simulink model "testbed_overall"  (R2022a)
settings: Solver=ode3  StartTime=0.0  StopTime=8  FixedStep=Ts  RelTol=1e-3
InitFcn:
  | f = 60;
  | Sb = 1e6; % base power
  | Vb_S = 13.2e3*sqrt(2)/sqrt(3);% secondary side base voltage phase to ground
  | Ib_S =Sb/Vb_S; % secondary side base current
  | Vb_P = 400*sqrt(2)/sqrt(3); % primary side base V
  | Ib_P = Sb/Vb_P; % primary side base I
  | Zb = ((400)^2)/Sb; % primary side base impedance
  | Zs = ((13.2e3)^2)/Sb; % secondary side base impedance
  | Zt = 0.02+1i*0.0721; % transformer impedance
  | Vg = 1;
  | P = 0.5;
  | Q = 0.5;
  | S = P+1i*Q;
  | I3 = conj(S/Vg);
  | V3 = Vg+I3*Zt; % pcc voltage in S side
  | % Vpcc = V3*Vb_S/Vb_P; % P side
  | Vpcc = V3;
  | R1 = 0.001/Zb;
  | L1 = (1i*120*pi*46e-6)/Zb; % impedacne ZL1
  | C1 = -(1i/(120*pi*3*444e-6))/Zb; %impedance ZC1
  | I2 = Vpcc/C1; % curreent going through the Capcitor
  | I1 = I2+I3;
  | V1 = Vpcc+I1*(R1+L1);
  | V = V1*Vb_P;
values from neighbouring files (symbols this model uses):
  ang_0 = 22*pi/180    (= 0.383972435439)    [GFM_initial.m]
  bc = w0*cf*zb1    (= 0.08034434716)    [GFM_initial.m]
  K1 = 1/0.05    (= 20)    [GFM_initial.m]
  K2 = 0.3    [GFM_initial.m]
  Ki_P = 25    [GFM_initial.m]
  ki_PLL = 1400    [GFM_initial.m]
  Ki_v = 40    [GFM_initial.m]
  Ki_vq = 10    [GFM_initial.m]
  kii = 3.2655    [GFM_initial.m]
  kiv = 40    [GFM_initial.m]
  Kp_P = 0.25    [GFM_initial.m]
  kp_PLL = 60    [GFM_initial.m]
  Kp_v = 0.4    [GFM_initial.m]
  Kp_vq = 1    [GFM_initial.m]
  kpi = 0.4758    [GFM_initial.m]
  kpv = 0.4    [GFM_initial.m]
  lg_real = xgrid_pu*zb2/w0    (= 0.369748763791)    [GFM_initial.m]
  rg_real = rgrid_pu*zb2    (= 13.9392)    [GFM_initial.m]
  Ts = 50e-6    (= 5e-05)    [GFM_initial.m]
  vb1 = vn1*sqrt(2/3)    [GFM_initial.m]
  w0 = 2*pi*f    (= 376.991118431)    [GFM_initial.m]
  xfpu = 2*pi*60*(46e-6)/0.16    (= 0.108384946549)    [GFM_initial.m]
undefined symbols (not defined in the file or in its folder): DiscIntNeverNeededParam
libraries: spsFirstOrderFilterLib x25, spsabctodq0Lib x13, spsPower3phInstantaneousLib x4, spsdq0toabcLib x4, spsThreePhaseVIMeasurementLib x4, spsThreePhaseSeriesRLCBranchLib x3, spsGroundLib x2, spsThreePhaseBreakerLib x2, spsSeriesRLCBranchLib x2, spsThreePhaseTransformerTwoWindingsLib x1, spsThreePhaseSeriesRLCLoadLib x1, spsThreePhaseParallelRLCBranchLib x1
settings Model: Creator=joshua  LastModifiedBy=PSCAD_FAN
settings SolverCC: AlgebraicLoopSolver=TrustRegion
settings DebuggingCC: UnconnectedInputMsg=warning  UnconnectedOutputMsg=warning  UnconnectedLineMsg=warning  SFMachineParentedDataDiag=warning  ArithmeticOperatorsInVariantConditions=warning
settings SFSimCC: CustomCodeUndefinedFunction=UseInterfaceOnly
settings RTWCC: DLArmComputeVersion=19.05
settings CodeAppCC: StateflowObjectComments=on
settings SimscapeCC: SimscapeNormalizeSystem=off

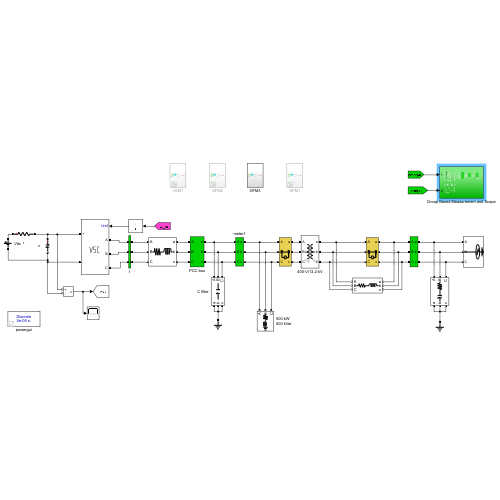
[thumbnail: Simulink's stored preview of the top-level diagram]
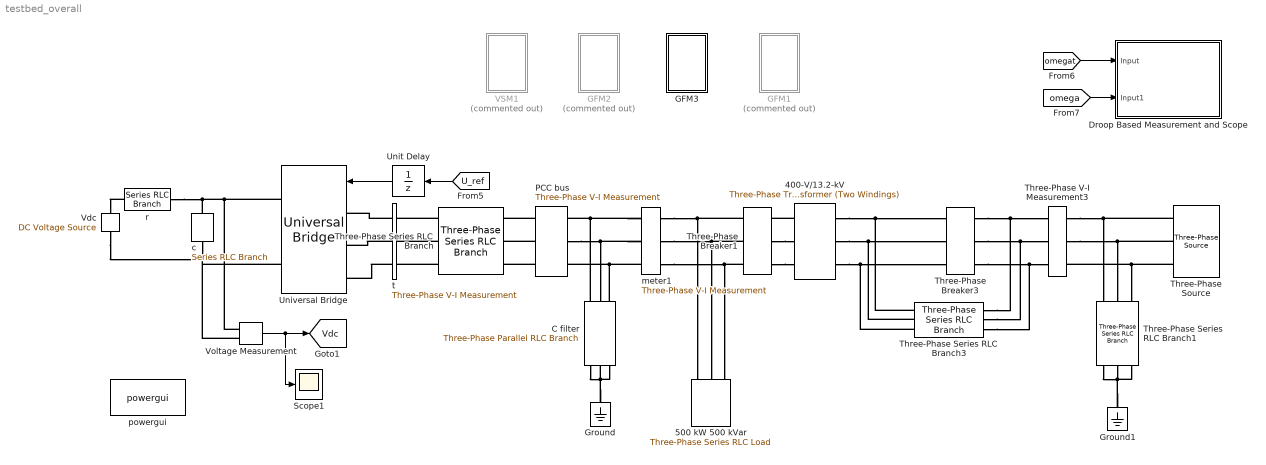
== system testbed_overall ==
  400-V/13.2-kV : spsThreePhaseTransformerTwoWindingsLib/Three-Phase Transformer (Two Windings)  Winding1Connection=Yg  Winding2Connection=Yg  CoreType=Three single-phase transformers  SetSaturation=off  Hysteresis=off  DataFile='hysteresis'  SetInitialFlux=off  Measurements=Winding voltages  UNITS=pu  NominalPower=[1e6 , 60 ]  Winding1=[400 0.01 0.0721/2]  Winding2=[13200 0.01 0.0721/2]  Rm=500  Lm=500  L0=0.50001  Saturation=[0 0;4.8989 1.0396;2041.2 1.3168]  InitialFluxes=[0.69306 -0.69306 0.60643]  BreakLoop=off  DiscreteSolver=Trapezoidal iterative  DataType=off  TransfoNumber=1
  500 kW 500 kVar : spsThreePhaseSeriesRLCLoadLib/Three-Phase Series RLC Load  LConnTagsString=A|B|C  Configuration=Y (grounded)  NominalVoltage=400  Vabc=[1e3 1e3 1e3]  Vabcp=[1e3 1e3 1e3]  NominalFrequency=f  UnbalancedPower=off  ActivePower=0.5*Sb  InductivePower=0.5*Sb  CapacitivePower=0  Pabc=[10e3 9e3 11e3]  QLabc=[100 90 110]  QCabc=[100 90 110]  Pabcp=[10e3 9e3 11e3]  QLabcp=[100 90 110]  QCabcp=[100 90 110]  Measurements=None  LoadType=constant Z
  C filter : spsThreePhaseParallelRLCBranchLib/Three-Phase Parallel RLC Branch  LConnTagsString=A|B|C  RConnTagsString=A|B|C  BranchType=C  Resistance=1  Inductance=1e-3  Capacitance=444e-6  Measurements=None
      settings: SourceProductBaseCode=PS
  Droop Based Measurement and Scope : Subsystem
  GFM1 : Subsystem  Commented=on
  GFM2 : Subsystem  Commented=on
  GFM3 : Subsystem
  Ground : spsGroundLib/Ground  LConnTagsString=a
  Ground1 : spsGroundLib/Ground  LConnTagsString=a
  PCC bus : spsThreePhaseVIMeasurementLib/Three-Phase V-I Measurement  VoltageMeasurement=phase-to-ground  SetLabelV=on  LabelV=Vpcc  Vpu=on  VpuLL=off  CurrentMeasurement=yes  SetLabelI=on  LabelI=Iconv  Ipu=on  Pbase=1e6  Vbase=400  OutputType=Complex  PhasorSimulation=off  PSBequivalent=0
  Scope1 : Scope
  Three-Phase Series RLC Branch : spsThreePhaseSeriesRLCBranchLib/Three-Phase Series RLC Branch  LConnTagsString=A|B|C  RConnTagsString=A|B|C  BranchType=RL  Resistance=0.001  Inductance=46e-6  Capacitance=1e-6  Measurements=None
  Three-Phase Series RLC Branch1 : spsThreePhaseSeriesRLCBranchLib/Three-Phase Series RLC Branch  LConnTagsString=A|B|C  RConnTagsString=A|B|C  BranchType=RC  Resistance=15  Inductance=1e-3  Capacitance=6.39e-6  Measurements=None
  Three-Phase Series RLC Branch3 : spsThreePhaseSeriesRLCBranchLib/Three-Phase Series RLC Branch  LConnTagsString=A|B|C  RConnTagsString=A|B|C  BranchType=RL  Resistance=rg_real  Inductance=lg_real  Capacitance=1e-6  Measurements=None
  Three-Phase V-I Measurement3 : spsThreePhaseVIMeasurementLib/Three-Phase V-I Measurement  VoltageMeasurement=phase-to-ground  SetLabelV=on  LabelV=Vabc  Vpu=on  VpuLL=off  CurrentMeasurement=yes  SetLabelI=on  LabelI=Ig  Ipu=on  Pbase=1e6  Vbase=13.2e3  OutputType=Complex  PhasorSimulation=off  PSBequivalent=0
  Three-Phase Breaker1 : spsThreePhaseBreakerLib/Three-Phase Breaker  InitialState=closed  SwitchA=on  SwitchB=on  SwitchC=on  SwitchTimes=[4,6]  External=off  BreakerResistance=0.0001  SnubberResistance=1e7  SnubberCapacitance=inf  Measurements=None
  Three-Phase Breaker3 : spsThreePhaseBreakerLib/Three-Phase Breaker  InitialState=closed  SwitchA=on  SwitchB=on  SwitchC=on  SwitchTimes=[2]  External=off  BreakerResistance=0.0001  SnubberResistance=1e7  SnubberCapacitance=inf  Measurements=None
  Three-Phase Source : spsThreePhaseSourceLib/Three-Phase Source  InternalConnection=Yg  VoltagePhases=off  Voltage=13.2e3  PhaseAngle=0  Voltage_phases=[25e3*0.5 25e3 25e3]/sqrt(3)  PhaseAngles_phases=[0 -120 +120]  Frequency=60  NonIdealSource=off  SpecifyImpedance=off  Resistance=0.8929  Inductance=16.58e-3  ShortCircuitLevel=100e6  BaseVoltage=25e3  XRratio=7  BusType=swing  Pref=10e3  Qref=0  Prefabc=[10e3, 10e3, 10e3]  Qrefabc=[0, 0, 0]  Qmin=-inf  Qmax=inf
  Unit Delay : UnitDelay  SampleTime=-1  HasFrameUpgradeWarning=on
  Universal Bridge : spsUniversalBridgeLib/Universal Bridge  Arms=3  SnubberResistance=1e5  SnubberCapacitance=inf  Device=Average-model based VSC  Ron=1e-3  Lon=0  ForwardVoltages="[  0  0  ]"  ForwardVoltage=0  GTOparameters=[ 10e-6 , 20e-6 ]  IGBTparameters=[ 1e-6 , 2e-6 ]  Measurements=None  Measurements_2=None  converterType=Rectifier
  VSM1 : Subsystem  Commented=on
  Vdc : spsDCVoltageSourceLib/DC Voltage Source  Amplitude=1025.6315  Measurements=None
  Voltage Measurement : spsVoltageMeasurementLib/Voltage Measurement  PhasorSimulation=off  OutputType=Complex  PSBequivalent=0
  c : spsSeriesRLCBranchLib/Series RLC Branch  LConnTagsString=__new0  RConnTagsString=__new0  BranchType=C  Resistance=0.05  Inductance=1e-3  SetiL0=off  InitialCurrent=0  Capacitance=0.04  Setx0=off  InitialVoltage=0  Measurements=Branch voltage
  meter1 : spsThreePhaseVIMeasurementLib/Three-Phase V-I Measurement  VoltageMeasurement=phase-to-ground  SetLabelV=on  LabelV=Vload  Vpu=on  VpuLL=off  CurrentMeasurement=yes  SetLabelI=on  LabelI=Iload  Ipu=on  Pbase=1e6  Vbase=400  OutputType=Complex  PhasorSimulation=off  PSBequivalent=0
  powergui : spspowerguiLib/powergui  Priority=1  SimulationMode=Discrete  SampleTime=50e-6  frequency=60  Iterations=50  frequencyindice=0  Pbase=100e6  ErrMax=1e-4  UnitsV=kV  UnitsW=MW  buscounter=0  FunctionMessages=off  echomessages=off  EnableUseOfTLC=off  CurrentSourceSwitches=off  DisableSnubberDevices=off  DisableRonSwitches=off  DisableVfSwitches=off  DisplayEquations=off  AutomaticDiscreteSolvers=off  SolverType=Tustin/Backward Euler (TBE)  Interpol=off  ExternalGateDelay=off  methode=off  Ts=100  x0status=blocks  SPID=on  SwTol=0  HookPort=off  NonlinearTolerance=1e-4  nMaxIteration=100  ContinueOnMaxIteration=off  RestoreLinks=warning  ResistiveCurrentMeasurement=off  Frange=[0:2:500]  Ylog=off  Xlog=on  ShowGrid=off  save=off  variable=ZData  structure=0  ZoomFFT=off  StartTime=0.0  cycles=1  DisplayStyle=1  fundamental=60  FreqAxis=off  MaxFrequency=1000  frequencyindicesteady=1  RmsSteady=1  display=off
  r : spsSeriesRLCBranchLib/Series RLC Branch  LConnTagsString=__new0  RConnTagsString=__new0  BranchType=R  Resistance=0.05  Inductance=1e-3  SetiL0=off  InitialCurrent=0  Capacitance=1e-6  Setx0=off  InitialVoltage=0  Measurements=None
  t : spsThreePhaseVIMeasurementLib/Three-Phase V-I Measurement  VoltageMeasurement=phase-to-ground  SetLabelV=on  LabelV=Vabc_o  Vpu=on  VpuLL=off  CurrentMeasurement=yes  SetLabelI=on  LabelI=Io  Ipu=on  Pbase=1e6  Vbase=400  OutputType=Complex  PhasorSimulation=off  PSBequivalent=0
  tag scope: Vdc=global
  wires:
  Voltage Measurement/1 -> Scope1/1, [Vdc]
  [U_ref] -> Unit Delay/1
  Unit Delay/1 -> Universal Bridge/1
  [omegat] -> Droop Based Measurement and Scope/1(Input)
  [omega] -> Droop Based Measurement and Scope/2(Input1)
  connections:
  Three-Phase Series RLC Branch1/RConn1 -- Three-Phase Series RLC Branch1/RConn3 -- Ground1/LConn1 -- Three-Phase Series RLC Branch1/RConn2
  PCC bus/RConn2 -- meter1/LConn2 -- C filter/LConn2
  Three-Phase V-I Measurement3/RConn2 -- Three-Phase Source/RConn2 -- Three-Phase Series RLC Branch1/LConn2
  Three-Phase Breaker1/LConn3 -- meter1/RConn3 -- 500 kW 500 kVar/LConn3
  Voltage Measurement/LConn1 -- Universal Bridge/RConn1 -- r/RConn1 -- c/LConn1
  c/RConn1 -- Universal Bridge/RConn2 -- Voltage Measurement/LConn2 -- Vdc/LConn1
  C filter/RConn2 -- C filter/RConn3 -- Ground/LConn1 -- C filter/RConn1
  C filter/LConn1 -- PCC bus/RConn1 -- meter1/LConn1
  Three-Phase V-I Measurement3/RConn1 -- Three-Phase Source/RConn1 -- Three-Phase Series RLC Branch1/LConn1
  Three-Phase Source/RConn3 -- Three-Phase V-I Measurement3/RConn3 -- Three-Phase Series RLC Branch1/LConn3
  400-V/13.2-kV/LConn1 -- Three-Phase Breaker1/RConn1
  r/LConn1 -- Vdc/RConn1
  Three-Phase Breaker1/RConn2 -- 400-V/13.2-kV/LConn2
  PCC bus/LConn3 -- Three-Phase Series RLC Branch/RConn3
  PCC bus/LConn1 -- Three-Phase Series RLC Branch/RConn1
  Three-Phase Series RLC Branch/LConn1 -- t/RConn1
  Three-Phase Breaker1/RConn3 -- 400-V/13.2-kV/LConn3
  t/LConn1 -- Universal Bridge/LConn1
  Three-Phase Series RLC Branch/LConn3 -- t/RConn3
  t/LConn2 -- Universal Bridge/LConn2
  PCC bus/LConn2 -- Three-Phase Series RLC Branch/RConn2
  t/LConn3 -- Universal Bridge/LConn3
  Three-Phase Series RLC Branch/LConn2 -- t/RConn2
  C filter/LConn3 -- meter1/LConn3 -- PCC bus/RConn3
  Three-Phase Breaker1/LConn2 -- meter1/RConn2 -- 500 kW 500 kVar/LConn2
  Three-Phase Breaker1/LConn1 -- meter1/RConn1 -- 500 kW 500 kVar/LConn1
  400-V/13.2-kV/RConn1 -- Three-Phase Series RLC Branch3/LConn1 -- Three-Phase Breaker3/LConn1
  400-V/13.2-kV/RConn2 -- Three-Phase Series RLC Branch3/LConn2 -- Three-Phase Breaker3/LConn2
  400-V/13.2-kV/RConn3 -- Three-Phase Series RLC Branch3/LConn3 -- Three-Phase Breaker3/LConn3
  Three-Phase Breaker3/RConn1 -- Three-Phase Series RLC Branch3/RConn1 -- Three-Phase V-I Measurement3/LConn1
  Three-Phase Breaker3/RConn2 -- Three-Phase V-I Measurement3/LConn2 -- Three-Phase Series RLC Branch3/RConn2
  Three-Phase Breaker3/RConn3 -- Three-Phase Series RLC Branch3/RConn3 -- Three-Phase V-I Measurement3/LConn3

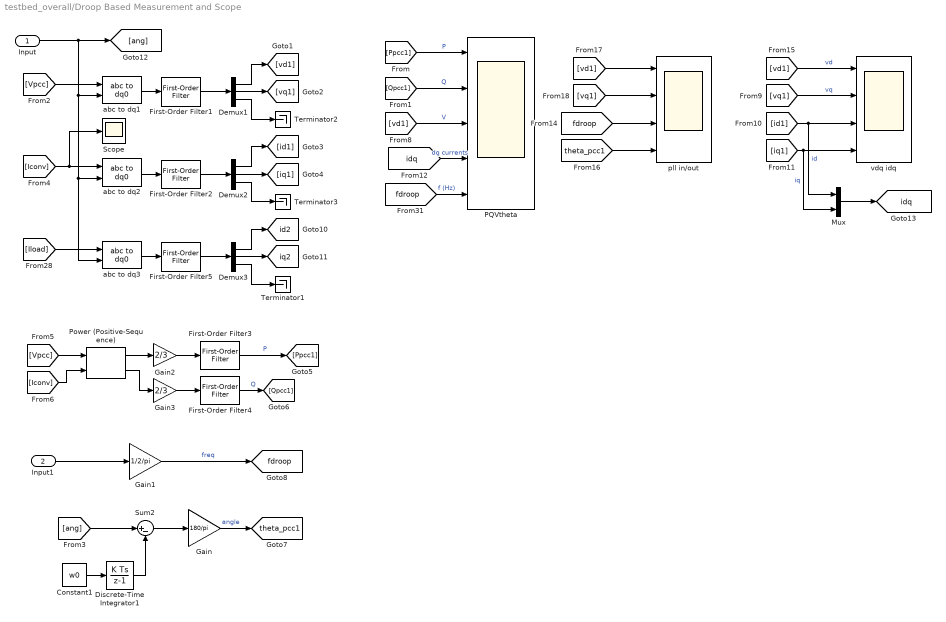
== system testbed_overall/Droop Based Measurement and Scope ==
  Input : Inport
  Input1 : Inport  Port=2
  Constant1 : Constant  Value=w0
  Demux1 : Demux  Outputs=3
  Demux2 : Demux  Outputs=3
  Demux3 : Demux  Outputs=3
  Discrete-Time Integrator1 : DiscreteIntegrator  SampleTime=Ts  ICPrevOutput=DiscIntNeverNeededParam  ICPrevScaledInput=DiscIntNeverNeededParam
  First-Order Filter{1..5} (5 alike) : spsFirstOrderFilterLib/First-Order Filter  FilterType=Lowpass  Tc=Tc  Ts=Ts  Initialize=off  Vac_Init=[0, 0, 60]  Vdc_Init=0  PlotResponse=off  FreqRange="[0,  200,  1]"
  Gain : Gain  Gain=180/pi
  Gain1 : Gain  Gain=1/2/pi
  Gain2 : Gain  Gain=2/3
  Gain3 : Gain  Gain=2/3
  Mux : Mux  Inputs=2
  PQVtheta : Scope  NumInputPorts=5
  Power (Positive-Sequence) : spsPowerPositiveSequenceLib/Power (Positive-Sequence)  Freq=60  Vinit=[0, 0]  Iinit=[0, 0]  Ts=0
      settings: SourceProductBaseCode=PS
  Scope : Scope
  Sum2 : Sum  Inputs=|+-
  Terminator1 : Terminator
  Terminator2 : Terminator
  Terminator3 : Terminator
  abc to dq1 : spsabctodq0Lib/abc to dq0  Alignment=90 degrees behind phase A axis
  abc to dq2 : spsabctodq0Lib/abc to dq0  Alignment=90 degrees behind phase A axis
  abc to dq3 : spsabctodq0Lib/abc to dq0  Alignment=90 degrees behind phase A axis
  pll in/out : Scope  NumInputPorts=4
  vdq idq : Scope  NumInputPorts=4
  tag scope: fdroop=global, id2=global, idq=global, iq2=global, theta_pcc1=global
  wires:
  [vd1] -> pll in/out/1
  [vd1] -> PQVtheta/3  "V"
  [iq1] -> Mux/2, vdq idq/4  "iq"
  [id1] -> Mux/1, vdq idq/3  "id"
  [theta_pcc1] -> pll in/out/4
  [vd1] -> vdq idq/1  "vd"
  [fdroop] -> pll in/out/3
  [vq1] -> vdq idq/2  "vq"
  [vq1] -> pll in/out/2
  [Ppcc1] -> PQVtheta/1  "P"
  [Qpcc1] -> PQVtheta/2  "Q"
  Gain1/1 -> [fdroop]  "freq"
  Gain/1 -> [theta_pcc1]  "angle"
  Sum2/1 -> Gain/1
  abc to dq1/1 -> First-Order Filter1/1
  Demux1/3 -> Terminator2/1
  abc to dq2/1 -> First-Order Filter2/1
  Discrete-Time Integrator1/1 -> Sum2/2
  Power (Positive-Sequence)/2 -> Gain3/1
  [ang] -> Sum2/1
  [Vpcc] -> abc to dq1/1
  [Vpcc] -> Power (Positive-Sequence)/1
  [Iconv] -> Power (Positive-Sequence)/2
  First-Order Filter3/1 -> [Ppcc1]  "P"
  Gain3/1 -> First-Order Filter4/1
  Gain2/1 -> First-Order Filter3/1
  Demux1/2 -> [vq1]
  Demux2/1 -> [id1]
  First-Order Filter4/1 -> [Qpcc1]  "Q"
  First-Order Filter1/1 -> Demux1/1
  [Iconv] -> Scope/1, abc to dq2/1
  First-Order Filter2/1 -> Demux2/1
  Power (Positive-Sequence)/1 -> Gain2/1
  Constant1/1 -> Discrete-Time Integrator1/1
  Demux2/3 -> Terminator3/1
  Demux2/2 -> [iq1]
  Demux1/1 -> [vd1]
  Demux3/2 -> [iq2]
  Input/1 -> [ang], abc to dq1/2, abc to dq3/2, abc to dq2/2
  Demux3/3 -> Terminator1/1
  First-Order Filter5/1 -> Demux3/1
  [Iload] -> abc to dq3/1
  Demux3/1 -> [id2]
  abc to dq3/1 -> First-Order Filter5/1
  Input1/1 -> Gain1/1
  Mux/1 -> [idq]
  [idq] -> PQVtheta/4  "dq currents"
  [fdroop] -> PQVtheta/5  "f (Hz)"

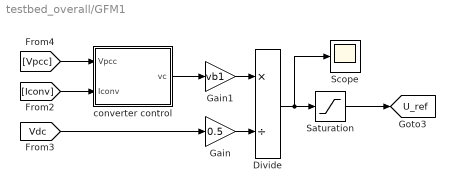
== system testbed_overall/GFM1 ==
  Divide : Product  Inputs=*/
  Gain : Gain  Gain=0.5
  Gain1 : Gain  Gain=vb1
  Saturation : Saturate  UpperLimit=1  LowerLimit=-1
  Scope : Scope
  converter control : Subsystem
  tag scope: U_ref=global
  wires:
  [Iconv] -> converter control/2(Iconv)
  Gain/1 -> Divide/2
  Saturation/1 -> [U_ref]
  [Vpcc] -> converter control/1(Vpcc)
  Gain1/1 -> Divide/1
  Divide/1 -> Scope/1, Saturation/1
  converter control/1(vc) -> Gain1/1
  [Vdc] -> Gain/1

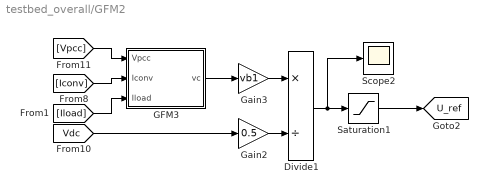
== system testbed_overall/GFM2 ==
  Divide1 : Product  Inputs=*/
  GFM3 : Subsystem
  Gain2 : Gain  Gain=0.5
  Gain3 : Gain  Gain=vb1
  Saturation1 : Saturate  UpperLimit=1  LowerLimit=-1
  Scope2 : Scope
  tag scope: U_ref=global
  wires:
  [Iconv] -> GFM3/2(Iconv)
  Gain2/1 -> Divide1/2
  GFM3/1(vc) -> Gain3/1
  [Vdc] -> Gain2/1
  Divide1/1 -> Scope2/1, Saturation1/1
  [Vpcc] -> GFM3/1(Vpcc)
  Gain3/1 -> Divide1/1
  Saturation1/1 -> [U_ref]
  [Iload] -> GFM3/3(Iload)

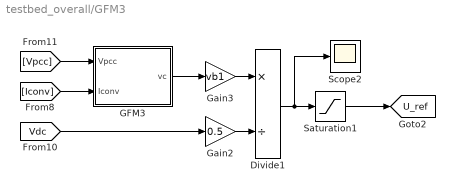
== system testbed_overall/GFM3 ==
  Divide1 : Product  Inputs=*/
  GFM3 : Subsystem
  Gain2 : Gain  Gain=0.5
  Gain3 : Gain  Gain=vb1
  Saturation1 : Saturate  UpperLimit=1  LowerLimit=-1
  Scope2 : Scope
  tag scope: U_ref=global
  wires:
  [Iconv] -> GFM3/2(Iconv)
  Gain2/1 -> Divide1/2
  GFM3/1(vc) -> Gain3/1
  [Vdc] -> Gain2/1
  Divide1/1 -> Scope2/1, Saturation1/1
  [Vpcc] -> GFM3/1(Vpcc)
  Gain3/1 -> Divide1/1
  Saturation1/1 -> [U_ref]

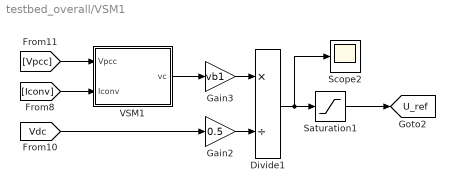
== system testbed_overall/VSM1 ==
  Divide1 : Product  Inputs=*/
  Gain2 : Gain  Gain=0.5
  Gain3 : Gain  Gain=vb1
  Saturation1 : Saturate  UpperLimit=1  LowerLimit=-1
  Scope2 : Scope
  VSM1 : Subsystem
  tag scope: U_ref=global
  wires:
  [Iconv] -> VSM1/2(Iconv)
  Gain2/1 -> Divide1/2
  VSM1/1(vc) -> Gain3/1
  [Vdc] -> Gain2/1
  Divide1/1 -> Scope2/1, Saturation1/1
  [Vpcc] -> VSM1/1(Vpcc)
  Gain3/1 -> Divide1/1
  Saturation1/1 -> [U_ref]

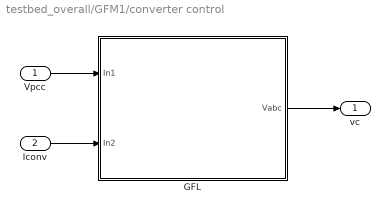
== system testbed_overall/GFM1/converter control ==
  Vpcc : Inport
  Iconv : Inport  Port=2
  GFL : Subsystem
  vc : Outport
  wires:
  Vpcc/1 -> GFL/1(In1)
  Iconv/1 -> GFL/2(In2)
  GFL/1(Vabc) -> vc/1

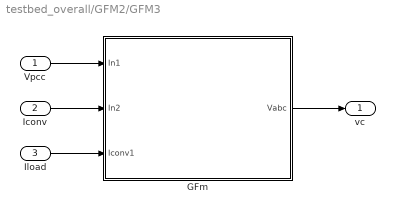
== system testbed_overall/GFM2/GFM3 ==
  Vpcc : Inport
  Iconv : Inport  Port=2
  Iload : Inport  Port=3
  GFm : Subsystem
  vc : Outport
  wires:
  Vpcc/1 -> GFm/1(In1)
  Iconv/1 -> GFm/2(In2)
  GFm/1(Vabc) -> vc/1
  Iload/1 -> GFm/3(Iconv1)

== system testbed_overall/GFM3/GFM3 ==
  Vpcc : Inport
  Iconv : Inport  Port=2
  GFm : Subsystem
  vc : Outport
  wires:
  Vpcc/1 -> GFm/1(In1)
  Iconv/1 -> GFm/2(In2)
  GFm/1(Vabc) -> vc/1

== system testbed_overall/VSM1/VSM1 ==
  Vpcc : Inport
  Iconv : Inport  Port=2
  VSM1 : Subsystem
  vc : Outport
  wires:
  Vpcc/1 -> VSM1/1(In1)
  Iconv/1 -> VSM1/2(In2)
  VSM1/1(Vabc) -> vc/1

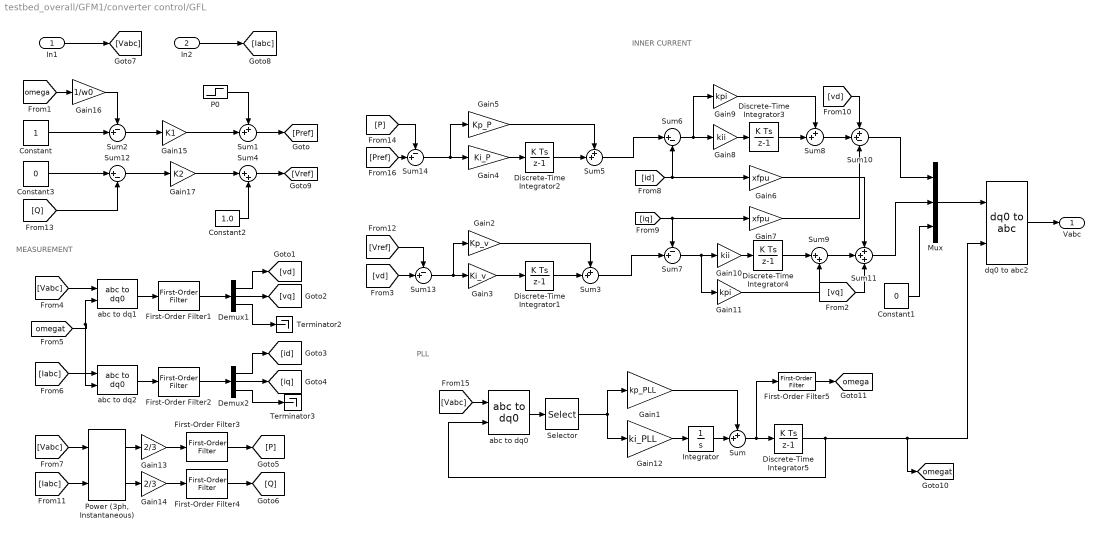
== system testbed_overall/GFM1/converter control/GFL ==
  note: PLL
  note: MEASUREMENT
  note: INNER
      | CURRENT
  In1 : Inport
  In2 : Inport  Port=2
  Constant : Constant
  Constant1 : Constant  Value=0
  Constant2 : Constant  Value=1.0
  Constant3 : Constant  Value=0
  Demux1 : Demux  Outputs=3
  Demux2 : Demux  Outputs=3
  Discrete-Time Integrator{1..5} (5 alike) : DiscreteIntegrator  SampleTime=Ts  ICPrevOutput=DiscIntNeverNeededParam  ICPrevScaledInput=DiscIntNeverNeededParam
  First-Order Filter{1..5} (5 alike) : spsFirstOrderFilterLib/First-Order Filter  FilterType=Lowpass  Tc=Tc  Ts=Ts  Initialize=off  Vac_Init=[0, 0, 60]  Vdc_Init=0  PlotResponse=off  FreqRange="[0,  200,  1]"
  Gain1 : Gain  Gain=kp_PLL
  Gain10 : Gain  Gain=kii
  Gain11 : Gain  Gain=kpi
  Gain12 : Gain  Gain=ki_PLL
  Gain13 : Gain  Gain=2/3
  Gain14 : Gain  Gain=2/3
  Gain15 : Gain  Gain=K1
  Gain16 : Gain  Gain=1/w0
  Gain17 : Gain  Gain=K2
  Gain2 : Gain  Gain=Kp_v
  Gain3 : Gain  Gain=Ki_v
  Gain4 : Gain  Gain=Ki_P
  Gain5 : Gain  Gain=Kp_P
  Gain6 : Gain  Gain=xfpu
  Gain7 : Gain  Gain=xfpu
  Gain8 : Gain  Gain=kii
  Gain9 : Gain  Gain=kpi
  Integrator : Integrator  InitialCondition=377
  Mux : Mux  Inputs=3
  P0 : Step  Before=0.1  SampleTime=0
  "Power (3ph, Instantaneous)" : spsPower3phInstantaneousLib/Power (3ph, Instantaneous)
  Selector : Selector  InputPortWidth=3  IndexOptions=Index vector (dialog)  Indices=[2]  OutputSizes=1
  Sum{,1,3,5,8} (5 alike) : Sum  Inputs=++|
  Sum10 : Sum  Inputs=++-
  Sum11 : Sum  Inputs=+++
  Sum12 : Sum  Inputs=|+-
  Sum{2,7,13..14} (4 alike) : Sum  Inputs=-+|
  Sum4 : Sum  Inputs=|++
  Sum6 : Sum  Inputs=|+-
  Sum9 : Sum  Inputs=|++
  Terminator2 : Terminator
  Terminator3 : Terminator
  abc to dq0 : spsabctodq0Lib/abc to dq0  Alignment=90 degrees behind phase A axis
  abc to dq1 : spsabctodq0Lib/abc to dq0  Alignment=90 degrees behind phase A axis
  abc to dq2 : spsabctodq0Lib/abc to dq0  Alignment=90 degrees behind phase A axis
  dq0 to abc2 : spsdq0toabcLib/dq0 to abc  Alignment=90 degrees behind phase A axis
  Vabc : Outport
  tag scope: omega=global, omegat=global
  wires:
  abc to dq2/1 -> First-Order Filter2/1
  [Pref] -> Sum14/2
  Gain3/1 -> Discrete-Time Integrator1/1
  Sum6/1 -> Gain8/1, Gain9/1
  [Vabc] -> "Power (3ph, Instantaneous)"/1
  Sum11/1 -> Mux/2
  Sum13/1 -> Gain3/1, Gain2/1
  Sum7/1 -> Gain11/1, Gain10/1
  "Power (3ph, Instantaneous)"/2 -> Gain14/1
  Constant1/1 -> Mux/3
  In2/1 -> [Iabc]
  Discrete-Time Integrator4/1 -> Sum9/1
  Gain5/1 -> Sum5/1
  [Vref] -> Sum13/1
  [Iabc] -> "Power (3ph, Instantaneous)"/2
  Sum14/1 -> Gain5/1, Gain4/1
  Sum3/1 -> Sum7/2
  Gain10/1 -> Discrete-Time Integrator4/1
  [id] -> Sum6/2, Gain6/1
  [omegat] -> abc to dq1/2, abc to dq2/2
  Sum8/1 -> Sum10/2
  Discrete-Time Integrator1/1 -> Sum3/2
  Demux1/3 -> Terminator2/1
  Gain2/1 -> Sum3/1
  Gain9/1 -> Sum8/1
  Discrete-Time Integrator3/1 -> Sum8/2
  Sum9/1 -> Sum11/2
  Gain4/1 -> Discrete-Time Integrator2/1
  First-Order Filter1/1 -> Demux1/1
  Gain8/1 -> Discrete-Time Integrator3/1
  [iq] -> Sum7/1, Gain7/1
  dq0 to abc2/1 -> Vabc/1
  Gain14/1 -> First-Order Filter4/1
  Gain11/1 -> Sum9/2
  Gain13/1 -> First-Order Filter3/1
  Sum10/1 -> Mux/1
  [vd] -> Sum13/2
  Demux1/1 -> [vd]
  Gain7/1 -> Sum10/3
  Gain6/1 -> Sum11/1
  [P] -> Sum14/1
  [Iabc] -> abc to dq2/1
  [Vabc] -> abc to dq1/1
  [vd] -> Sum10/1
  Mux/1 -> dq0 to abc2/1
  Demux2/3 -> Terminator3/1
  abc to dq1/1 -> First-Order Filter1/1
  Demux2/1 -> [id]
  In1/1 -> [Vabc]
  Discrete-Time Integrator2/1 -> Sum5/2
  First-Order Filter3/1 -> [P]
  First-Order Filter2/1 -> Demux2/1
  Sum5/1 -> Sum6/1
  Demux1/2 -> [vq]
  Demux2/2 -> [iq]
  First-Order Filter4/1 -> [Q]
  "Power (3ph, Instantaneous)"/1 -> Gain13/1
  Discrete-Time Integrator5/1 -> abc to dq0/2, dq0 to abc2/2, [omegat]
  [vq] -> Sum11/3
  Integrator/1 -> Sum/2
  Gain1/1 -> Sum/1
  Gain12/1 -> Integrator/1
  [Vabc] -> abc to dq0/1
  abc to dq0/1 -> Selector/1
  Selector/1 -> Gain12/1, Gain1/1
  Sum/1 -> First-Order Filter5/1, Discrete-Time Integrator5/1
  P0/1 -> Sum1/1
  Sum1/1 -> [Pref]
  Sum2/1 -> Gain15/1
  Gain16/1 -> Sum2/1
  Constant/1 -> Sum2/2
  [omega] -> Gain16/1
  Sum4/1 -> [Vref]
  Constant2/1 -> Sum4/2
  Sum12/1 -> Gain17/1
  Constant3/1 -> Sum12/1
  [Q] -> Sum12/2
  First-Order Filter5/1 -> [omega]
  Gain15/1 -> Sum1/2
  Gain17/1 -> Sum4/1

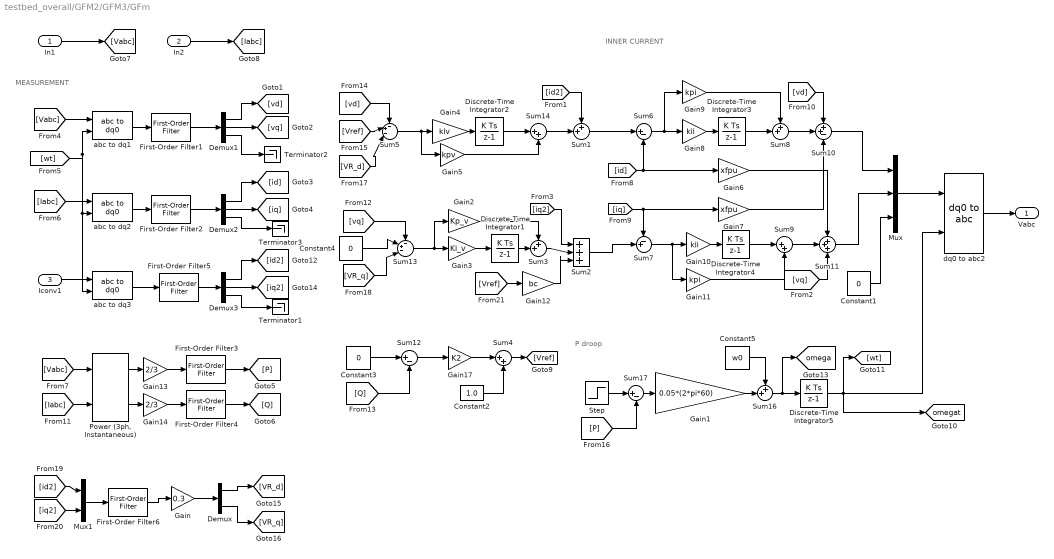
== system testbed_overall/GFM2/GFM3/GFm ==
  note: MEASUREMENT
  note: INNER
      | CURRENT
  note: P droop
  In1 : Inport
  In2 : Inport  Port=2
  Iconv1 : Inport  Port=3
  Constant1 : Constant  Value=0
  Constant2 : Constant  Value=1.0
  Constant3 : Constant  Value=0
  Constant4 : Constant  Value=0
  Constant5 : Constant  Value=w0
  Demux : Demux  Outputs=2
  Demux1 : Demux  Outputs=3
  Demux2 : Demux  Outputs=3
  Demux3 : Demux  Outputs=3
  Discrete-Time Integrator{1..4} (4 alike) : DiscreteIntegrator  SampleTime=Ts  ICPrevOutput=DiscIntNeverNeededParam  ICPrevScaledInput=DiscIntNeverNeededParam
  Discrete-Time Integrator5 : DiscreteIntegrator  InitialCondition=ang_0*0  SampleTime=Ts  ICPrevOutput=DiscIntNeverNeededParam  ICPrevScaledInput=DiscIntNeverNeededParam
  First-Order Filter{1..5} (5 alike) : spsFirstOrderFilterLib/First-Order Filter  FilterType=Lowpass  Tc=Tc  Ts=Ts  Initialize=off  Vac_Init=[0, 0, 60]  Vdc_Init=0  PlotResponse=off  FreqRange="[0,  200,  1]"
  First-Order Filter6 : spsFirstOrderFilterLib/First-Order Filter  FilterType=Highpass  Tc=0.1  Ts=Ts  Initialize=off  Vac_Init=[0, 0, 60]  Vdc_Init=0  PlotResponse=off  FreqRange="[0,  200,  1]"
  Gain : Gain  Gain=0.3
  Gain1 : Gain  Gain=0.05*(2*pi*60)
  Gain10 : Gain  Gain=kii
  Gain11 : Gain  Gain=kpi
  Gain12 : Gain  Gain=bc
  Gain13 : Gain  Gain=2/3
  Gain14 : Gain  Gain=2/3
  Gain17 : Gain  Gain=K2
  Gain2 : Gain  Gain=Kp_v
  Gain3 : Gain  Gain=Ki_v
  Gain4 : Gain  Gain=kiv
  Gain5 : Gain  Gain=kpv
  Gain6 : Gain  Gain=xfpu
  Gain7 : Gain  Gain=xfpu
  Gain8 : Gain  Gain=kii
  Gain9 : Gain  Gain=kpi
  Mux : Mux  Inputs=3
  Mux1 : Mux  Inputs=2
  "Power (3ph, Instantaneous)" : spsPower3phInstantaneousLib/Power (3ph, Instantaneous)
  Step : Step  SampleTime=0
  Sum{1,3,8,16} (4 alike) : Sum  Inputs=++|
  Sum10 : Sum  Inputs=++-
  Sum11 : Sum  Inputs=+++
  Sum12 : Sum  Inputs=|+-
  Sum13 : Sum  Inputs=-+-|
  Sum14 : Sum  Inputs=|++
  Sum17 : Sum  Inputs=|+-
  Sum2 : Sum  Inputs=+++|
  Sum4 : Sum  Inputs=|++
  Sum5 : Sum  Inputs=-+-|
  Sum6 : Sum  Inputs=|+-
  Sum7 : Sum  Inputs=-+|
  Sum9 : Sum  Inputs=|++
  Terminator1 : Terminator
  Terminator2 : Terminator
  Terminator3 : Terminator
  abc to dq1 : spsabctodq0Lib/abc to dq0  Alignment=90 degrees behind phase A axis
  abc to dq2 : spsabctodq0Lib/abc to dq0  Alignment=90 degrees behind phase A axis
  abc to dq3 : spsabctodq0Lib/abc to dq0  Alignment=90 degrees behind phase A axis
  dq0 to abc2 : spsdq0toabcLib/dq0 to abc  Alignment=90 degrees behind phase A axis
  Vabc : Outport
  tag scope: omega=global, omegat=global
  wires:
  abc to dq2/1 -> First-Order Filter2/1
  Gain3/1 -> Discrete-Time Integrator1/1
  Sum6/1 -> Gain8/1, Gain9/1
  [Vabc] -> "Power (3ph, Instantaneous)"/1
  Sum11/1 -> Mux/2
  Sum13/1 -> Gain3/1, Gain2/1
  Sum7/1 -> Gain11/1, Gain10/1
  "Power (3ph, Instantaneous)"/2 -> Gain14/1
  Constant1/1 -> Mux/3
  In2/1 -> [Iabc]
  Discrete-Time Integrator4/1 -> Sum9/1
  [vq] -> Sum13/1
  [Iabc] -> "Power (3ph, Instantaneous)"/2
  Gain10/1 -> Discrete-Time Integrator4/1
  [id] -> Sum6/2, Gain6/1
  Sum8/1 -> Sum10/2
  Discrete-Time Integrator1/1 -> Sum3/2
  Demux1/3 -> Terminator2/1
  Gain2/1 -> Sum3/1
  Gain9/1 -> Sum8/1
  Discrete-Time Integrator3/1 -> Sum8/2
  Sum9/1 -> Sum11/2
  First-Order Filter1/1 -> Demux1/1
  Gain8/1 -> Discrete-Time Integrator3/1
  [iq] -> Sum7/1, Gain7/1
  dq0 to abc2/1 -> Vabc/1
  Gain14/1 -> First-Order Filter4/1
  Gain11/1 -> Sum9/2
  Gain13/1 -> First-Order Filter3/1
  Sum10/1 -> Mux/1
  Constant4/1 -> Sum13/2
  Demux1/1 -> [vd]
  Gain7/1 -> Sum10/3
  Gain6/1 -> Sum11/1
  [Iabc] -> abc to dq2/1
  [Vabc] -> abc to dq1/1
  [vd] -> Sum10/1
  Mux/1 -> dq0 to abc2/1
  Demux2/3 -> Terminator3/1
  abc to dq1/1 -> First-Order Filter1/1
  Demux2/1 -> [id]
  In1/1 -> [Vabc]
  First-Order Filter3/1 -> [P]
  First-Order Filter2/1 -> Demux2/1
  Demux1/2 -> [vq]
  Demux2/2 -> [iq]
  First-Order Filter4/1 -> [Q]
  "Power (3ph, Instantaneous)"/1 -> Gain13/1
  [vq] -> Sum11/3
  Sum4/1 -> [Vref]
  Constant2/1 -> Sum4/2
  Sum12/1 -> Gain17/1
  Constant3/1 -> Sum12/1
  [Q] -> Sum12/2
  [vd] -> Sum5/1
  [Vref] -> Sum5/2
  Sum5/1 -> Gain5/1, Gain4/1
  Discrete-Time Integrator2/1 -> Sum14/1
  Gain5/1 -> Sum14/2
  Gain4/1 -> Discrete-Time Integrator2/1
  Constant5/1 -> Sum16/1
  Discrete-Time Integrator5/1 -> [omegat], dq0 to abc2/2, [wt]
  Sum16/1 -> [omega], Discrete-Time Integrator5/1
  Gain1/1 -> Sum16/2
  Sum17/1 -> Gain1/1
  [P] -> Sum17/2
  Step/1 -> Sum17/1
  Sum14/1 -> Sum1/2
  Sum1/1 -> Sum6/1
  Sum2/1 -> Sum7/2
  Sum3/1 -> Sum2/2
  Iconv1/1 -> abc to dq3/1
  Demux3/3 -> Terminator1/1
  abc to dq3/1 -> First-Order Filter5/1
  Demux3/1 -> [id2]
  [wt] -> abc to dq1/2, abc to dq3/2, abc to dq2/2
  Demux3/2 -> [iq2]
  Gain17/1 -> Sum4/1
  First-Order Filter5/1 -> Demux3/1
  [id2] -> Sum1/1
  [iq2] -> Sum2/1
  [VR_d] -> Sum5/3
  [VR_q] -> Sum13/3
  [id2] -> Mux1/1
  [iq2] -> Mux1/2
  Mux1/1 -> First-Order Filter6/1
  First-Order Filter6/1 -> Gain/1
  Gain/1 -> Demux/1
  Demux/1 -> [VR_d]
  Demux/2 -> [VR_q]
  [Vref] -> Gain12/1
  Gain12/1 -> Sum2/3

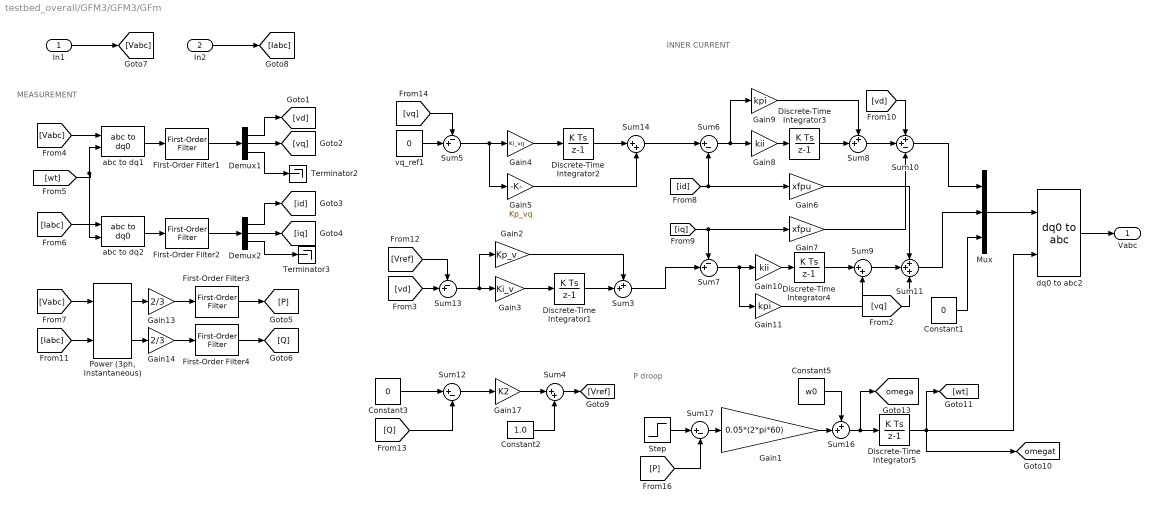
== system testbed_overall/GFM3/GFM3/GFm ==
  note: MEASUREMENT
  note: INNER
      | CURRENT
  note: P droop
  In1 : Inport
  In2 : Inport  Port=2
  Constant1 : Constant  Value=0
  Constant2 : Constant  Value=1.0
  Constant3 : Constant  Value=0
  Constant5 : Constant  Value=w0
  Demux1 : Demux  Outputs=3
  Demux2 : Demux  Outputs=3
  Discrete-Time Integrator{1..4} (4 alike) : DiscreteIntegrator  SampleTime=Ts  ICPrevOutput=DiscIntNeverNeededParam  ICPrevScaledInput=DiscIntNeverNeededParam
  Discrete-Time Integrator5 : DiscreteIntegrator  InitialCondition=ang_0*0  SampleTime=Ts  ICPrevOutput=DiscIntNeverNeededParam  ICPrevScaledInput=DiscIntNeverNeededParam
  First-Order Filter{1..4} (4 alike) : spsFirstOrderFilterLib/First-Order Filter  FilterType=Lowpass  Tc=Tc  Ts=Ts  Initialize=off  Vac_Init=[0, 0, 60]  Vdc_Init=0  PlotResponse=off  FreqRange="[0,  200,  1]"
  Gain1 : Gain  Gain=0.05*(2*pi*60)
  Gain10 : Gain  Gain=kii
  Gain11 : Gain  Gain=kpi
  Gain13 : Gain  Gain=2/3
  Gain14 : Gain  Gain=2/3
  Gain17 : Gain  Gain=K2
  Gain2 : Gain  Gain=Kp_v
  Gain3 : Gain  Gain=Ki_v
  Gain4 : Gain  Gain=Ki_vq
  Gain5 : Gain  Gain=Kp_vq
  Gain6 : Gain  Gain=xfpu
  Gain7 : Gain  Gain=xfpu
  Gain8 : Gain  Gain=kii
  Gain9 : Gain  Gain=kpi
  Mux : Mux  Inputs=3
  "Power (3ph, Instantaneous)" : spsPower3phInstantaneousLib/Power (3ph, Instantaneous)
  Step : Step  SampleTime=0
  Sum10 : Sum  Inputs=++-
  Sum11 : Sum  Inputs=+++
  Sum12 : Sum  Inputs=|+-
  Sum13 : Sum  Inputs=-+|
  Sum14 : Sum  Inputs=|++
  Sum16 : Sum  Inputs=++|
  Sum17 : Sum  Inputs=|+-
  Sum3 : Sum  Inputs=++|
  Sum4 : Sum  Inputs=|++
  Sum5 : Sum  Inputs=-+|
  Sum6 : Sum  Inputs=|+-
  Sum7 : Sum  Inputs=-+|
  Sum8 : Sum  Inputs=++|
  Sum9 : Sum  Inputs=|++
  Terminator2 : Terminator
  Terminator3 : Terminator
  abc to dq1 : spsabctodq0Lib/abc to dq0  Alignment=90 degrees behind phase A axis
  abc to dq2 : spsabctodq0Lib/abc to dq0  Alignment=90 degrees behind phase A axis
  dq0 to abc2 : spsdq0toabcLib/dq0 to abc  Alignment=90 degrees behind phase A axis
  vq_ref1 : Constant  Value=0
  Vabc : Outport
  tag scope: omega=global, omegat=global
  wires:
  abc to dq2/1 -> First-Order Filter2/1
  Gain3/1 -> Discrete-Time Integrator1/1
  Sum6/1 -> Gain8/1, Gain9/1
  [Vabc] -> "Power (3ph, Instantaneous)"/1
  Sum11/1 -> Mux/2
  Sum13/1 -> Gain3/1, Gain2/1
  Sum7/1 -> Gain11/1, Gain10/1
  "Power (3ph, Instantaneous)"/2 -> Gain14/1
  Constant1/1 -> Mux/3
  In2/1 -> [Iabc]
  Discrete-Time Integrator4/1 -> Sum9/1
  [Vref] -> Sum13/1
  [Iabc] -> "Power (3ph, Instantaneous)"/2
  Sum3/1 -> Sum7/2
  Gain10/1 -> Discrete-Time Integrator4/1
  [id] -> Sum6/2, Gain6/1
  [wt] -> abc to dq1/2, abc to dq2/2
  Sum8/1 -> Sum10/2
  Discrete-Time Integrator1/1 -> Sum3/2
  Demux1/3 -> Terminator2/1
  Gain2/1 -> Sum3/1
  Gain9/1 -> Sum8/1
  Discrete-Time Integrator3/1 -> Sum8/2
  Sum9/1 -> Sum11/2
  First-Order Filter1/1 -> Demux1/1
  Gain8/1 -> Discrete-Time Integrator3/1
  [iq] -> Sum7/1, Gain7/1
  dq0 to abc2/1 -> Vabc/1
  Gain14/1 -> First-Order Filter4/1
  Gain11/1 -> Sum9/2
  Gain13/1 -> First-Order Filter3/1
  Sum10/1 -> Mux/1
  [vd] -> Sum13/2
  Demux1/1 -> [vd]
  Gain7/1 -> Sum10/3
  Gain6/1 -> Sum11/1
  [Iabc] -> abc to dq2/1
  [Vabc] -> abc to dq1/1
  [vd] -> Sum10/1
  Mux/1 -> dq0 to abc2/1
  Demux2/3 -> Terminator3/1
  abc to dq1/1 -> First-Order Filter1/1
  Demux2/1 -> [id]
  In1/1 -> [Vabc]
  First-Order Filter3/1 -> [P]
  First-Order Filter2/1 -> Demux2/1
  Demux1/2 -> [vq]
  Demux2/2 -> [iq]
  First-Order Filter4/1 -> [Q]
  "Power (3ph, Instantaneous)"/1 -> Gain13/1
  [vq] -> Sum11/3
  Sum4/1 -> [Vref]
  Constant2/1 -> Sum4/2
  Sum12/1 -> Gain17/1
  Constant3/1 -> Sum12/1
  [Q] -> Sum12/2
  Gain17/1 -> Sum4/1
  [vq] -> Sum5/1
  Sum14/1 -> Sum6/1
  vq_ref1/1 -> Sum5/2
  Sum5/1 -> Gain5/1, Gain4/1
  Discrete-Time Integrator2/1 -> Sum14/1
  Gain5/1 -> Sum14/2
  Gain4/1 -> Discrete-Time Integrator2/1
  Constant5/1 -> Sum16/1
  Discrete-Time Integrator5/1 -> [omegat], dq0 to abc2/2, [wt]
  Sum16/1 -> [omega], Discrete-Time Integrator5/1
  Gain1/1 -> Sum16/2
  Sum17/1 -> Gain1/1
  [P] -> Sum17/2
  Step/1 -> Sum17/1

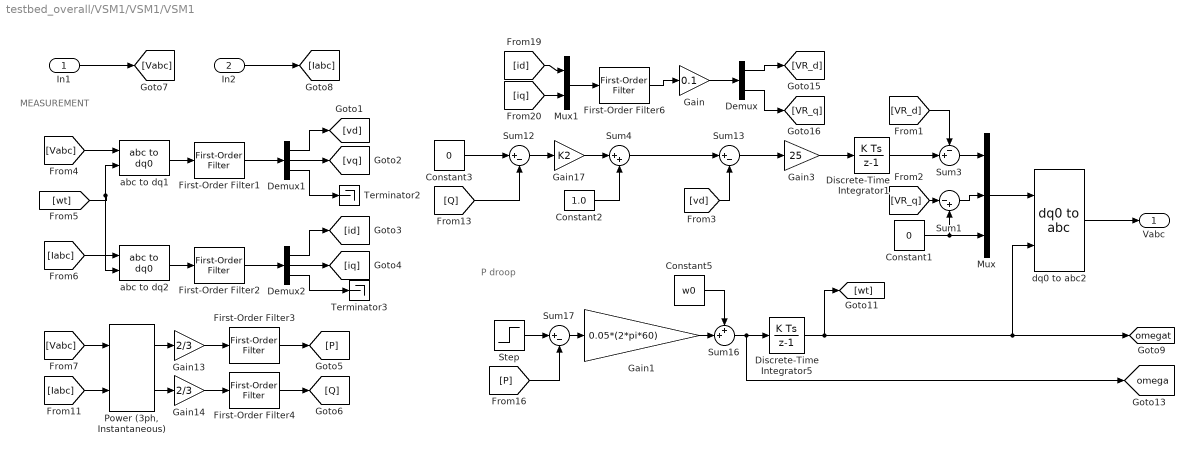
== system testbed_overall/VSM1/VSM1/VSM1 ==
  note: MEASUREMENT
  note: P droop
  In1 : Inport
  In2 : Inport  Port=2
  Constant1 : Constant  Value=0
  Constant2 : Constant  Value=1.0
  Constant3 : Constant  Value=0
  Constant5 : Constant  Value=w0
  Demux : Demux  Outputs=2
  Demux1 : Demux  Outputs=3
  Demux2 : Demux  Outputs=3
  Discrete-Time Integrator1 : DiscreteIntegrator  SampleTime=Ts  ICPrevOutput=DiscIntNeverNeededParam  ICPrevScaledInput=DiscIntNeverNeededParam
  Discrete-Time Integrator5 : DiscreteIntegrator  InitialCondition=ang_0*0  SampleTime=Ts  ICPrevOutput=DiscIntNeverNeededParam  ICPrevScaledInput=DiscIntNeverNeededParam
  First-Order Filter{1..4} (4 alike) : spsFirstOrderFilterLib/First-Order Filter  FilterType=Lowpass  Tc=Tc  Ts=Ts  Initialize=off  Vac_Init=[0, 0, 60]  Vdc_Init=0  PlotResponse=off  FreqRange="[0,  200,  1]"
  First-Order Filter6 : spsFirstOrderFilterLib/First-Order Filter  FilterType=Highpass  Tc=0.1  Ts=Ts  Initialize=off  Vac_Init=[0, 0, 60]  Vdc_Init=0  PlotResponse=off  FreqRange="[0,  200,  1]"
  Gain : Gain  Gain=0.1
  Gain1 : Gain  Gain=0.05*(2*pi*60)
  Gain13 : Gain  Gain=2/3
  Gain14 : Gain  Gain=2/3
  Gain17 : Gain  Gain=K2
  Gain3 : Gain  Gain=25
  Mux : Mux  Inputs=3
  Mux1 : Mux  Inputs=2
  "Power (3ph, Instantaneous)" : spsPower3phInstantaneousLib/Power (3ph, Instantaneous)
  Step : Step  SampleTime=0
  Sum1 : Sum  Inputs=|-+
  Sum12 : Sum  Inputs=|+-
  Sum13 : Sum  Inputs=|+-
  Sum16 : Sum  Inputs=++|
  Sum17 : Sum  Inputs=|+-
  Sum3 : Sum  Inputs=-+|
  Sum4 : Sum  Inputs=|++
  Terminator2 : Terminator
  Terminator3 : Terminator
  abc to dq1 : spsabctodq0Lib/abc to dq0  Alignment=90 degrees behind phase A axis
  abc to dq2 : spsabctodq0Lib/abc to dq0  Alignment=90 degrees behind phase A axis
  dq0 to abc2 : spsdq0toabcLib/dq0 to abc  Alignment=90 degrees behind phase A axis
  Vabc : Outport
  tag scope: omega=global, omegat=global
  wires:
  abc to dq2/1 -> First-Order Filter2/1
  Gain3/1 -> Discrete-Time Integrator1/1
  [Vabc] -> "Power (3ph, Instantaneous)"/1
  Sum13/1 -> Gain3/1
  "Power (3ph, Instantaneous)"/2 -> Gain14/1
  Constant1/1 -> Mux/3, Sum1/2
  In2/1 -> [Iabc]
  [Iabc] -> "Power (3ph, Instantaneous)"/2
  [wt] -> abc to dq1/2, abc to dq2/2
  Discrete-Time Integrator1/1 -> Sum3/2
  Demux1/3 -> Terminator2/1
  First-Order Filter1/1 -> Demux1/1
  dq0 to abc2/1 -> Vabc/1
  Gain14/1 -> First-Order Filter4/1
  Gain13/1 -> First-Order Filter3/1
  Demux1/1 -> [vd]
  [Iabc] -> abc to dq2/1
  [Vabc] -> abc to dq1/1
  Mux/1 -> dq0 to abc2/1
  Demux2/3 -> Terminator3/1
  abc to dq1/1 -> First-Order Filter1/1
  Demux2/1 -> [id]
  In1/1 -> [Vabc]
  First-Order Filter3/1 -> [P]
  First-Order Filter2/1 -> Demux2/1
  Demux1/2 -> [vq]
  Demux2/2 -> [iq]
  First-Order Filter4/1 -> [Q]
  "Power (3ph, Instantaneous)"/1 -> Gain13/1
  Sum4/1 -> Sum13/1
  Constant2/1 -> Sum4/2
  Sum12/1 -> Gain17/1
  Constant3/1 -> Sum12/1
  [Q] -> Sum12/2
  Gain17/1 -> Sum4/1
  Constant5/1 -> Sum16/1
  Discrete-Time Integrator5/1 -> [omegat], dq0 to abc2/2, [wt]
  Sum16/1 -> [omega], Discrete-Time Integrator5/1
  Gain1/1 -> Sum16/2
  Sum17/1 -> Gain1/1
  [P] -> Sum17/2
  Step/1 -> Sum17/1
  [vd] -> Sum13/2
  Sum3/1 -> Mux/1
  Demux/2 -> [VR_q]
  Gain/1 -> Demux/1
  [id] -> Mux1/1
  [iq] -> Mux1/2
  Demux/1 -> [VR_d]
  First-Order Filter6/1 -> Gain/1
  Mux1/1 -> First-Order Filter6/1
  Sum1/1 -> Mux/2
  [VR_d] -> Sum3/1
  [VR_q] -> Sum1/1
